simulink model "carsim_test2017"  (R2017b)
settings: Solver=FixedStepAuto  StartTime=0.0  StopTime=20  FixedStep=0.001  RelTol=1e-3
undefined symbols (not defined in the file or in its folder): ACC_MAP, ACC_MAP_ACCPEDL_BPY, ACC_MAP_REFSPD_BPX, BRK_MAP, BRK_MAP_BRKPEDL_BPX, ConvGear, CORNERING_STIFFNESS_APT, DIST_FR_AXLE_TO_CG_NVV, DIST_RE_AXLE_TO_CG_NVV, Fz, Fz_BPX, geartar, HYD_RATIO_APT, HYDRATIO_REFSPD_BPX, REFSPD_Q, REFSPD_R_LGT, REFSPD_R_WHL, STATIC_SPD, STATIC_TIME, VEHICLE_MASS_NVV, VEHICLE_YAW_INERTIA_NVV
libraries: simulink x22, simulink_extras x2, Solver_SF x1, SignalEditorBlockLib x1
(part 2 of 2)

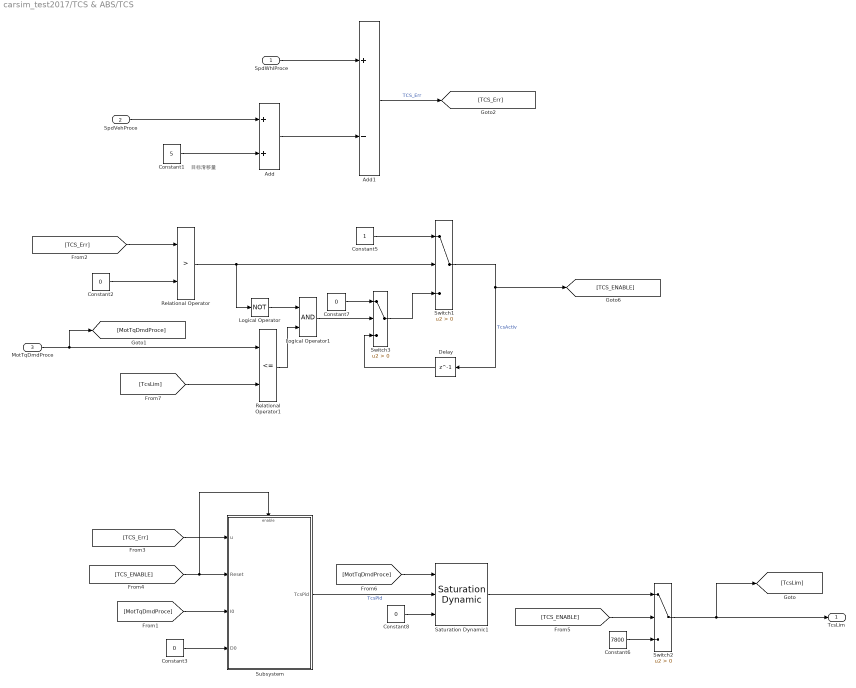
== system carsim_test2017/TCS & ABS/TCS ==
  note: 目标滑移量
  SpdWhlProce : Inport
  SpdVehProce : Inport  Port=2
  MotTqDmdProce : Inport  Port=3
  Add : Sum
  Add1 : Sum  Inputs=+-
  Constant1 : Constant  Value=5
  Constant{2..3,7..8} (4 alike) : Constant  Value=0
  Constant5 : Constant
  Constant6 : Constant  Value=7800
  Delay : Delay  DelayLength=1
  Logical Operator : Logic  Operator=NOT  AllPortsSameDT=off  OutDataTypeStr=boolean
  Logical Operator1 : Logic  AllPortsSameDT=off  OutDataTypeStr=boolean
  Relational Operator : RelationalOperator  Operator=>  OutDataTypeStr=boolean  RndMeth=Simplest
  Relational Operator1 : RelationalOperator  Operator=<=  OutDataTypeStr=boolean  RndMeth=Simplest
  Saturation Dynamic1 : simulink/Discontinuities/Saturation Dynamic  OutMin=[]  OutMax=[]  OutDataTypeStr=Inherit: Same as second input  OutDataType=fixdt(1, 16)  OutScaling=2^-10  DoSatur=off
  Subsystem : Subsystem
  Switch1 : Switch  Criteria=u2 > Threshold
  Switch2 : Switch  Criteria=u2 > Threshold
  Switch3 : Switch  Criteria=u2 > Threshold
  TcsLim : Outport
  wires:
  [TCS_Err] -> Subsystem/1(u)
  Constant5/1 -> Switch1/1
  Switch1/1 -> [TCS_ENABLE], Delay/1  "TcsActiv"
  [MotTqDmdProce] -> Saturation Dynamic1/1
  [TCS_ENABLE] -> Subsystem/Enable, Subsystem/2(Reset)
  Switch2/1 -> TcsLim/1, [TcsLim]
  Logical Operator/1 -> Logical Operator1/1
  Add/1 -> Add1/2
  [TcsLim] -> Relational Operator1/2
  Constant2/1 -> Relational Operator/2
  Switch3/1 -> Switch1/3
  Constant8/1 -> Saturation Dynamic1/3
  Logical Operator1/1 -> Switch3/2
  Add1/1 -> [TCS_Err]  "TCS_Err"
  Constant1/1 -> Add/2
  Delay/1 -> Switch3/3
  MotTqDmdProce/1 -> [MotTqDmdProce], Relational Operator1/1
  Relational Operator1/1 -> Logical Operator1/2
  Subsystem/1(TcsPid) -> Saturation Dynamic1/2  "TcsPid"
  Relational Operator/1 -> Logical Operator/1, Switch1/2
  SpdWhlProce/1 -> Add1/1
  [TCS_ENABLE] -> Switch2/2
  Constant7/1 -> Switch3/1
  [TCS_Err] -> Relational Operator/1
  Constant6/1 -> Switch2/3
  Saturation Dynamic1/1 -> Switch2/1
  [MotTqDmdProce] -> Subsystem/3(I0)
  Constant3/1 -> Subsystem/4(D0)
  SpdVehProce/1 -> Add/1

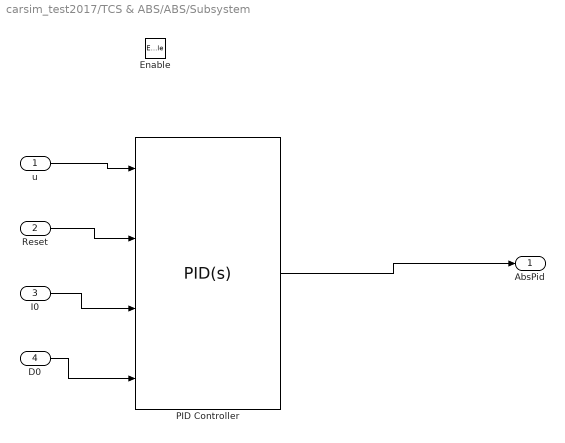
== system carsim_test2017/TCS & ABS/ABS/Subsystem ==
  u : Inport
  Reset : Inport  Port=2
  I0 : Inport  Port=3
  D0 : Inport  Port=4
  Enable : EnablePort  StatesWhenEnabling=reset
  PID Controller : simulink/Continuous/PID Controller  Controller=PID  Form=Parallel  TimeDomain=Continuous-time  SampleTime=-1  IntegratorMethod=Forward Euler  ControllerParametersSource=internal  P=100  I=500  D=0  N=100  UseFilter=on  TunerSelectOption=Transfer Function Based (PID Tuner App)  InitialConditionSource=external  InitialConditionForIntegrator=0  InitialConditionForFilter=0  DifferentiatorICPrevScaledInput=0  ExternalReset=either  TrackingMode=off  Kt=1  LimitOutput=off  UpperSaturationLimit=inf  LowerSaturationLimit=-inf  LinearizeAsGain=on  AntiWindupMode=none  Kb=1  POutMin=[]  POutMax=[]  IOutMin=[]  IOutMax=[]  DOutMin=[]  DOutMax=[]  NOutMin=[]  NOutMax=[]  SumOutMin=[]  SumOutMax=[]  SaturationOutMin=[]  SaturationOutMax=[]  PParamMin=[]  PParamMax=[]  IParamMin=[]  IParamMax=[]  DParamMin=[]  DParamMax=[]  NParamMin=[]  NParamMax=[]  KbParamMin=[]  KbParamMax=[]  KtParamMin=[]  KtParamMax=[]  KbOutMin=[]  KbOutMax=[]  KtOutMin=[]  KtOutMax=[]  IntegratorOutMin=[]  IntegratorOutMax=[]  FilterOutMin=[]  FilterOutMax=[]  SumI1OutMin=[]  SumI1OutMax=[]  SumI2OutMin=[]  SumI2OutMax=[]  SumI3OutMin=[]  SumI3OutMax=[]  SumDOutMin=[]  SumDOutMax=[]  DifferentiatorOutMin=[]  DifferentiatorOutMax=[]  FilterDiffOutCoefMin=[]  FilterDiffOutCoefMax=[]  ReciprocalOutMin=[]  ReciprocalOutMax=[]  SumDenOutMin=[]  SumDenOutMax=[]  SumNumOutMin=[]  SumNumOutMax=[]  DivideOutMin=[]  DivideOutMax=[]  IntegratorContinuousStateAttributes=''  IntegratorStateMustResolveToSignalObject=off  IntegratorRTWStateStorageClass=Auto  FilterContinuousStateAttributes=''  FilterStateMustResolveToSignalObject=off  FilterRTWStateStorageClass=Auto  InitialConditionSetting=State (most efficient)
  AbsPid : Outport  OutputWhenDisabled=reset  InitialOutput=-8000
  wires:
  Reset/1 -> PID Controller/2
  I0/1 -> PID Controller/3
  PID Controller/1 -> AbsPid/1
  u/1 -> PID Controller/1
  D0/1 -> PID Controller/4

== system carsim_test2017/TCS & ABS/TCS/Subsystem ==
  u : Inport
  Reset : Inport  Port=2
  I0 : Inport  Port=3
  D0 : Inport  Port=4
  Enable : EnablePort  StatesWhenEnabling=reset
  PID Controller : simulink/Continuous/PID Controller  Controller=PID  Form=Parallel  TimeDomain=Continuous-time  SampleTime=-1  IntegratorMethod=Forward Euler  ControllerParametersSource=internal  P=-100  I=-500  D=0  N=100  UseFilter=on  TunerSelectOption=Transfer Function Based (PID Tuner App)  InitialConditionSource=external  InitialConditionForIntegrator=0  InitialConditionForFilter=0  DifferentiatorICPrevScaledInput=0  ExternalReset=either  TrackingMode=off  Kt=1  LimitOutput=off  UpperSaturationLimit=inf  LowerSaturationLimit=-inf  LinearizeAsGain=on  AntiWindupMode=none  Kb=1  POutMin=[]  POutMax=[]  IOutMin=[]  IOutMax=[]  DOutMin=[]  DOutMax=[]  NOutMin=[]  NOutMax=[]  SumOutMin=[]  SumOutMax=[]  SaturationOutMin=[]  SaturationOutMax=[]  PParamMin=[]  PParamMax=[]  IParamMin=[]  IParamMax=[]  DParamMin=[]  DParamMax=[]  NParamMin=[]  NParamMax=[]  KbParamMin=[]  KbParamMax=[]  KtParamMin=[]  KtParamMax=[]  KbOutMin=[]  KbOutMax=[]  KtOutMin=[]  KtOutMax=[]  IntegratorOutMin=[]  IntegratorOutMax=[]  FilterOutMin=[]  FilterOutMax=[]  SumI1OutMin=[]  SumI1OutMax=[]  SumI2OutMin=[]  SumI2OutMax=[]  SumI3OutMin=[]  SumI3OutMax=[]  SumDOutMin=[]  SumDOutMax=[]  DifferentiatorOutMin=[]  DifferentiatorOutMax=[]  FilterDiffOutCoefMin=[]  FilterDiffOutCoefMax=[]  ReciprocalOutMin=[]  ReciprocalOutMax=[]  SumDenOutMin=[]  SumDenOutMax=[]  SumNumOutMin=[]  SumNumOutMax=[]  DivideOutMin=[]  DivideOutMax=[]  IntegratorContinuousStateAttributes=''  IntegratorStateMustResolveToSignalObject=off  IntegratorRTWStateStorageClass=Auto  FilterContinuousStateAttributes=''  FilterStateMustResolveToSignalObject=off  FilterRTWStateStorageClass=Auto  InitialConditionSetting=State (most efficient)
  TcsPid : Outport  OutputWhenDisabled=reset  InitialOutput=7800
  wires:
  D0/1 -> PID Controller/4
  u/1 -> PID Controller/1
  PID Controller/1 -> TcsPid/1
  I0/1 -> PID Controller/3
  Reset/1 -> PID Controller/2

== matlab function carsim_test2017/Subsystem/MATLAB Function1 ==
  data: a11 input; A output; a12 input; a21 input; a22 input
function A = fcn(a11, a12, a21, a22)
%#codegen
A = [a11, a12; a21, a22];
end

== matlab function carsim_test2017/Subsystem/MATLAB Function ==
  data: x input; dx output; u input; y output; A input; B input; C input; D input
function [dx, y] = state_space_derivative(x, u, A, B, C, D)
    % 计算连续时间状态导数
    dx = A * x + B * u;
    y  = C * x + D * u;
end

== matlab function carsim_test2017/Subsystem/MATLAB Function2 ==
  data: b11 input; B output; b21 input
function B = fcn(b11, b21)
%#codegen
B = [b11;b21];
end

== matlab function carsim_test2017/Subsystem/MATLAB Function3 ==
  data: a11 input; A output; a12 input; a21 input; a22 input
function A = fcn(a11, a12, a21, a22)
%#codegen
A = [a11, a12; a21, a22];
end

== matlab function carsim_test2017/Subsystem/MATLAB Function4 ==
  data: b11 input; B output; b21 input
function B = fcn(b11, b21)
%#codegen
B = [b11;b21];
end

== matlab function carsim_test2017/MATLAB Function ==
  data: a_meas input; omega_pitch input; v_wheel input; is_static input; dt input; Q input; R_wheel input; R_accel input; v output; b output; theta output; a output; P output
function [v, b, theta, a, P] = vehicleSpeedEKF4(a_meas, omega_pitch, v_wheel, is_static, dt, Q, R_wheel, R_accel)
% vehicleSpeedEKF4 - 四维EKF车速估计（增加真实加速度状态）
%
% 输入:
%   a_meas      - 纵向加速度计测量值 (m/s^2)
%   omega_pitch - 俯仰角速度 (rad/s)
%   v_wheel     - 轮速等效车速 (m/s)
%   is_static   - 静止标志 (true/false)
%   dt          - 采样时间 (s)
%   Q           - 过程噪声协方差 (4×4)
%   R_wheel     - 轮速观测噪声方差 (标量)
%   R_accel     - 加速度计观测噪声方差 (标量)
%
% 输出:
%   v, b, theta, a - 估计的状态
%   P             - 误差协方差矩阵 (4×4)
%
% 内部常量（可修改）：
%   R_STAT_V  - 静止时虚拟速度零观测噪声 (默认 1e-4)
%   R_STAT_A  - 静止时加速度计观测噪声 (默认 0.01)
%
% 重置滤波器: clear vehicleSpeedEKF4

    persistent x P_persistent
    g = 9.81;
    
    % 静止观测噪声（内部固定）
    R_STAT_V = 1e-6;
    R_STAT_A = 0.01;
    
    % 初始化
    if isempty(x)
        x = [0; 0; 0; 0];                     % [v; b; theta; a]
        P_persistent = diag([1, 0.1, 0.01, 1]); % 初始协方差
    end
    
    % ========== 预测 ==========
    v_prev = x(1); b_prev = x(2); theta_prev = x(3); a_prev = x(4);
    
    % 状态预测（非线性部分仅theta）
    v_pred   = v_prev + a_prev * dt;
    b_pred   = b_prev;
    theta_pred = theta_prev + omega_pitch * dt;
    a_pred   = a_prev;
    x_pred = [v_pred; b_pred; theta_pred; a_pred];
    
    % 雅可比矩阵 F (4×4)
    F = [1, 0, 0, dt;
         0, 1, 0, 0;
         0, 0, 1, 0;
         0, 0, 0, 1];
    
    P_pred = F * P_persistent * F' + Q;
    
    % ========== 更新 ==========
    if is_static
        % 静止：观测 [0; a_meas]
        z_pred = [v_pred; b_pred + g * sin(theta_pred)];
        z = [0; a_meas];
        H = [1, 0, 0, 0;
             0, 1, g*cos(theta_pred), 0];
        R = diag([R_STAT_V, R_STAT_A]);
    else
        % 运动：观测 [v_wheel; a_meas]
        z_pred = [v_pred; a_pred + b_pred + g * sin(theta_pred)];
        z = [v_wheel; a_meas];
        H = [1, 0, 0, 0;
             0, 1, g*cos(theta_pred), 1];
        R = diag([R_wheel, R_accel]);
    end
    
    % 卡尔曼更新
    y = z - z_pred;
    S = H * P_pred * H' + R;
    K = P_pred * H' / S;
    x = x_pred + K * y;
    P_persistent = (eye(4) - K * H) * P_pred;
    
    % 输出
    v = x(1);
    b = x(2);
    theta = x(3);
    a = x(4);
    P = P_persistent;
end

== matlab function carsim_test2017/Subsystem1/MATLAB Function ==
  data: slipFlags input; wheelSpeedOut output; wheelSpeeds input; allSlipFlag output
function [wheelSpeedOut, allSlipFlag] = computeWheelSpeed(slipFlags, wheelSpeeds)
%#codegen
% computeWheelSpeed: output mean of non-slip wheel speeds, or min if all slip.
%
% Inputs:
%   slipFlags   - slip indicator array (0 = no slip, nonzero = slip)
%   wheelSpeeds - wheel speed array (same number of elements as slipFlags)
%
% Outputs:
%   wheelSpeedOut - calculated wheel speed
%   allSlipFlag   - 1 (double) if all wheels are slipping, 0 (double) otherwise

    % Check that both inputs have the same total number of elements
    if numel(slipFlags) ~= numel(wheelSpeeds)
        error('slipFlags and wheelSpeeds must have the same number of elements.');
    end

    % Convert to logical array (0 -> false, nonzero -> true)
    slipLogical = logical(slipFlags);

    % Determine if all wheels are slipping, and store directly as double (0 or 1)
    % This avoids changing the variable type later, satisfying code generation.
    allSlipFlag = double(all(slipLogical(:)));

    if allSlipFlag
        % All wheels slip: output the minimum wheel speed
        wheelSpeedOut = min(wheelSpeeds(:));
    else
        % Some wheels not slipping: output mean of those speeds
        % Logical indexing uses linear order (column-major), works for any shape
        wheelSpeedOut = mean(wheelSpeeds(~slipLogical));
    end
end

== matlab function carsim_test2017/MATLAB Function1 ==
  data: u input; y output; Ts input; delay input
function y = turnOnDelay(u, Ts,  delay)
%#codegen
% turnOnDelay - Turn-on delay for multidimensional input (no partial assignment)
%
%   Inputs:
%       u     : current input (any dimension, nonzero = true)
%       Ts    : sample time in seconds (must be > 0)
%       delay : delay time in seconds (>= 0)
%   Output:
%       y     : delayed output (same size as u, double 0 or 1)

persistent timerCount lastInput output delaySteps

% ---------- Validate Ts ----------
if Ts <= 0
    error('Sample time Ts must be greater than 0.');
end

% ---------- Initialize persistent states ----------
if isempty(timerCount)
    timerCount = zeros(size(u));
    lastInput  = false(size(u));
    output     = false(size(u));
    delaySteps = max(0, round(delay / Ts));
else
    % If input size changes, reinitialize
    if ~isequal(size(timerCount), size(u))
        timerCount = zeros(size(u));
        lastInput  = false(size(u));
        output     = false(size(u));
        delaySteps = max(0, round(delay / Ts));
    end
end

% Update delay steps if parameters changed online
newSteps = max(0, round(delay / Ts));
if newSteps ~= delaySteps
    delaySteps = newSteps;
end

% ---------- Current input as logical ----------
currentInput = (u ~= 0);

% ---------- Detect edges ----------
rise = currentInput & ~lastInput;   % 0→1 transition
hold = currentInput & ~rise;        % stayed 1 (not just rose)

% ---------- Update per‑channel timers (completely index‑free) ----------
% Timer logic:
%   - on rising edge: reset to 0
%   - if input stays true: increment by 1
%   - if input false: reset to 0
% Arithmetic equivalent (elementwise):
%   timerCount = (timerCount .* ~rise + hold) .* currentInput;
% But we must also handle the case when delaySteps becomes 0 (no delay),
% then output should be true immediately for rising edge? Original behavior
% says: rising edge sets timer=0, and if delaySteps=0 output goes true only
% after one sample (because on the rising sample, output remains false).
% Our arithmetic does exactly that.

timerCount = (timerCount .* (~rise) + hold) .* currentInput;

% ---------- Compute output completely by elementwise logic ----------
% Output true only when input is true, NOT on the rising edge, and timer >= delaySteps.
% Since 'hold' already excludes the rising edge, we can simply use:
output = hold & (timerCount >= delaySteps);

% ---------- Store current input for next step ----------
lastInput = currentInput;

% ---------- Output ----------
y = double(output);
end

== matlab function carsim_test2017/Subsystem1/MATLAB Function1 ==
  data: u input; y output; Ts input; delay input
function y = turnOnDelay(u, Ts, delay)
%#codegen
% turnOnDelay - Turn-on delay for multidimensional input (no partial assignment)
%
%   Inputs:
%       u     : current input (any dimension, nonzero = true)
%       Ts    : sample time in seconds (must be > 0)
%       delay : delay time in seconds (>= 0)
%   Output:
%       y     : delayed output (same size as u, double 0 or 1)

persistent timerCount lastInput output delaySteps

% ---------- Validate Ts ----------
if Ts <= 0
    error('Sample time Ts must be greater than 0.');
end

% ---------- Initialize persistent states ----------
if isempty(timerCount)
    timerCount = zeros(size(u));
    lastInput  = false(size(u));
    output     = false(size(u));
    delaySteps = max(0, round(delay / Ts));
else
    % If input size changes, reinitialize
    if ~isequal(size(timerCount), size(u))
        timerCount = zeros(size(u));
        lastInput  = false(size(u));
        output     = false(size(u));
        delaySteps = max(0, round(delay / Ts));
    end
end

% Update delay steps if parameters changed online
newSteps = max(0, round(delay / Ts));
if newSteps ~= delaySteps
    delaySteps = newSteps;
end

% ---------- Current input as logical ----------
currentInput = (u ~= 0);

% ---------- Detect edges ----------
rise = currentInput & ~lastInput;   % 0→1 transition
hold = currentInput & ~rise;        % stayed 1 (not just rose)

% ---------- Update per‑channel timers (completely index‑free) ----------
% Timer logic:
%   - on rising edge: reset to 0
%   - if input stays true: increment by 1
%   - if input false: reset to 0
% Arithmetic equivalent (elementwise):
%   timerCount = (timerCount .* ~rise + hold) .* currentInput;
% But we must also handle the case when delaySteps becomes 0 (no delay),
% then output should be true immediately for rising edge? Original behavior
% says: rising edge sets timer=0, and if delaySteps=0 output goes true only
% after one sample (because on the rising sample, output remains false).
% Our arithmetic does exactly that.

timerCount = (timerCount .* (~rise) + hold) .* currentInput;

% ---------- Compute output completely by elementwise logic ----------
% Output true only when input is true, NOT on the rising edge, and timer >= delaySteps.
% Since 'hold' already excludes the rising edge, we can simply use:
output = hold & (timerCount >= delaySteps);

% ---------- Store current input for next step ----------
lastInput = currentInput;

% ---------- Output ----------
y = double(output);
end

== matlab function carsim_test2017/Subsystem1/MATLAB Function2 ==
  data: u input; y output; Ts input; delay input
function y = turnOnDelay(u, Ts, delay)
%#codegen
% turnOnDelay - Turn-on delay for multidimensional input (no partial assignment)
%
%   Inputs:
%       u     : current input (any dimension, nonzero = true)
%       Ts    : sample time in seconds (must be > 0)
%       delay : delay time in seconds (>= 0)
%   Output:
%       y     : delayed output (same size as u, double 0 or 1)

persistent timerCount lastInput output delaySteps

% ---------- Validate Ts ----------
if Ts <= 0
    error('Sample time Ts must be greater than 0.');
end

% ---------- Initialize persistent states ----------
if isempty(timerCount)
    timerCount = zeros(size(u));
    lastInput  = false(size(u));
    output     = false(size(u));
    delaySteps = max(0, round(delay / Ts));
else
    % If input size changes, reinitialize
    if ~isequal(size(timerCount), size(u))
        timerCount = zeros(size(u));
        lastInput  = false(size(u));
        output     = false(size(u));
        delaySteps = max(0, round(delay / Ts));
    end
end

% Update delay steps if parameters changed online
newSteps = max(0, round(delay / Ts));
if newSteps ~= delaySteps
    delaySteps = newSteps;
end

% ---------- Current input as logical ----------
currentInput = (u ~= 0);

% ---------- Detect edges ----------
rise = currentInput & ~lastInput;   % 0→1 transition
hold = currentInput & ~rise;        % stayed 1 (not just rose)

% ---------- Update per‑channel timers (completely index‑free) ----------
% Timer logic:
%   - on rising edge: reset to 0
%   - if input stays true: increment by 1
%   - if input false: reset to 0
% Arithmetic equivalent (elementwise):
%   timerCount = (timerCount .* ~rise + hold) .* currentInput;
% But we must also handle the case when delaySteps becomes 0 (no delay),
% then output should be true immediately for rising edge? Original behavior
% says: rising edge sets timer=0, and if delaySteps=0 output goes true only
% after one sample (because on the rising sample, output remains false).
% Our arithmetic does exactly that.

timerCount = (timerCount .* (~rise) + hold) .* currentInput;

% ---------- Compute output completely by elementwise logic ----------
% Output true only when input is true, NOT on the rising edge, and timer >= delaySteps.
% Since 'hold' already excludes the rising edge, we can simply use:
output = hold & (timerCount >= delaySteps);

% ---------- Store current input for next step ----------
lastInput = currentInput;

% ---------- Output ----------
y = double(output);
end

== matlab function carsim_test2017/MATLAB Function2 ==
  data: gyro input; accel input; v_wheel input; dt input; v_car output; slip_flag input; a_long output; pitch_deg output
function [v_car, a_long, pitch_deg] = estimateVelocity(gyro, accel, v_wheel, dt, slip_flag)
% 基于单轮速+IMU的车速估计（修正版：雅可比矩阵修正，四元数归一化）
% 输入：
%   gyro      : 车体系三轴角速度 [wx;wy;wz] (rad/s)
%   accel     : 车体系三轴加速度 [ax;ay;az] (m/s^2)
%   v_wheel   : 后轴（或单个）轮速线速度 (m/s)
%   dt        : 时间步长 (s)
%   slip_flag : 打滑标志，0=正常，1=轮速不可信（噪声极大）
% 输出：
%   v_car     : 估计的前向车速 (m/s)
%   a_long    : 纵向运动加速度（不含重力分量）(m/s^2)
%   pitch_deg : 俯仰角（上坡为正，度）

    persistent kf
    if isempty(kf)
        kf = initializeFilter();
    end

    x = kf.x;
    P = kf.P;
    dx = kf.dx;
    mem = kf.mem;
    cfg = kf.cfg;

    % ---------- 1. 预测 ----------
    gW = [0; 0; -cfg.g];
    b_g = x(11:13);
    b_a = x(14:16);
    gyro_ub  = gyro - b_g;
    accel_ub = accel - b_a;

    R_BW = quat2rot(x(7:10));
    dq = rotvec2quat(gyro_ub * dt);
    q_BW_new = quatMul(x(7:10), dq);
    q_BW_new = normalizeQuat(q_BW_new);  % 归一化
    R_new = quat2rot(q_BW_new);

    acc_world = R_BW * accel_ub + gW;
    v_W_new = x(4:6) + acc_world * dt;
    p_W_new = x(1:3) + x(4:6)*dt + 0.5*acc_world*dt^2;
    x_new = [p_W_new; v_W_new; q_BW_new; b_g; b_a];

    % ---------- 2. 协方差预测 ----------
    Omega_x = skew(gyro_ub);
    A_x = skew(accel_ub);
    F = zeros(15);
    F(1:3,1:3)   = -Omega_x;
    F(1:3,10:12) = -eye(3);
    F(4:6,1:3)   = -R_BW * A_x;
    F(4:6,13:15) = -R_BW;
    F(7:9,4:6)   = eye(3);

    G = zeros(15,12);
    G(1:3,1:3)   = -eye(3);
    G(4:6,4:6)   = -R_BW;
    G(10:12,7:9) = eye(3);
    G(13:15,10:12)= eye(3);

    Qc = blkdiag(cfg.sigma_g^2*eye(3), cfg.sigma_a^2*eye(3), ...
                 cfg.sigma_bg^2*eye(3), cfg.sigma_ba^2*eye(3));
    Phi = eye(15) + F * dt;
    P_new = Phi * P * Phi' + Phi * G * Qc * G' * Phi' * dt;

    % ---------- 3. 观测更新 ----------
    function injectAndReset()
        x_new(7:10) = quatMul(x_new(7:10), rotvec2quat(dx(1:3)));
        x_new(7:10) = normalizeQuat(x_new(7:10));
        x_new(4:6)  = x_new(4:6)  + dx(4:6);
        x_new(1:3)  = x_new(1:3)  + dx(7:9);
        x_new(11:13)= x_new(11:13)+ dx(10:12);
        x_new(14:16)= x_new(14:16)+ dx(13:15);
        dx = zeros(15,1);
        R_new = quat2rot(x_new(7:10));
        v_W_new = x_new(4:6);
    end

    % 预计算车体系速度和重力向量（雅可比修正依赖）
    v_body = R_new' * v_W_new;
    g_body = R_new' * gW;

    % 3.1 轮速观测
    h_vx = v_body(1);
    H_vx = zeros(1,15);
    % 修正：用 v_body 构造反对称矩阵的对应行
    H_vx(1:3) = [0, -v_body(3), v_body(2)];
    H_vx(4:6) = R_new(:,1)';

    if slip_flag
        R_vx = 1e6;
    else
        if mem.wheel_init && dt > 0
            a_wheel_est = (v_wheel - mem.last_v_wheel)/dt;
            % 注意：此处 a_imu_est 是车体系 x 向的运动加速度（世界加速度投影）
            a_imu_est   = R_new(:,1)' * (R_new * accel_ub + gW);
            slip_factor = abs(a_wheel_est - a_imu_est);
            R_vx = cfg.sigma_vx_base * exp(cfg.slip_gain * slip_factor);
        else
            R_vx = cfg.sigma_vx_base;
            mem.wheel_init = true;
        end
    end
    mem.last_v_wheel = v_wheel;

    [P_new, dx] = ekfUpdate(P_new, dx, v_wheel - h_vx, H_vx, R_vx);
    injectAndReset();
    % 更新后需重新计算 v_body（因为速度/姿态更新）
    v_body = R_new' * v_W_new;

    % 3.2 侧向约束 vy=0
    h_vy = v_body(2);
    H_vy = zeros(1,15);
    H_vy(1:3) = [v_body(3), 0, -v_body(1)];
    H_vy(4:6) = R_new(:,2)';
    yaw_rate = gyro(3);
    if mem.yaw_init && dt > 0
        % 注意：侧滑检测逻辑可能需按车辆动力学修正，这里保留原逻辑框架
        slip_lat = abs((yaw_rate - mem.last_yaw_rate)/dt + accel(2));
    else
        slip_lat = 0;
        mem.yaw_init = true;
    end
    mem.last_yaw_rate = yaw_rate;
    R_vy = cfg.sigma_vy_base * exp(cfg.slip_gain_vy * slip_lat);
    [P_new, dx] = ekfUpdate(P_new, dx, 0 - h_vy, H_vy, R_vy);
    injectAndReset();
    v_body = R_new' * v_W_new;

    % 3.3 垂向约束 vz=0
    h_vz = v_body(3);
    H_vz = zeros(1,15);
    H_vz(1:3) = [-v_body(2), v_body(1), 0];
    H_vz(4:6) = R_new(:,3)';
    [P_new, dx] = ekfUpdate(P_new, dx, 0 - h_vz, H_vz, cfg.sigma_vz);
    injectAndReset();
    v_body = R_new' * v_W_new;
    g_body = R_new' * gW;

    % 3.4 重力对准
    if abs(norm(accel) - cfg.g) < cfg.grav_acc_thresh && norm(gyro) < cfg.grav_gyro_thresh
        z_grav = accel;
        h_grav = -g_body + x_new(14:16);
        H_grav = zeros(3,15);
        % 修正：使用 skew(g_body) 作为姿态误差的雅可比
        H_grav(1:3,1:3)   = skew(g_body);
        H_grav(1:3,13:15) = eye(3);
        [P_new, dx] = ekfUpdate(P_new, dx, z_grav - h_grav, H_grav, cfg.sigma_grav^2*eye(3));
        injectAndReset();
        v_body = R_new' * v_W_new;  % 不需要 g_body，但保持一致
    end

    % 3.5 零速更新
    if abs(v_wheel) < cfg.zupt_wheel_thresh && ...
       norm(accel - mem.last_accel) < cfg.zupt_accel_variation
        z_zupt = zeros(3,1);
        h_zupt = v_W_new;
        H_zupt = zeros(3,15);
        H_zupt(1:3,4:6) = eye(3);
        [P_new, dx] = ekfUpdate(P_new, dx, z_zupt - h_zupt, H_zupt, cfg.sigma_zupt^2*eye(3));
        injectAndReset();
    end
    mem.last_accel = accel;

    % ---------- 4. 保存状态 ----------
    kf.x = x_new;
    kf.P = P_new;
    kf.dx = dx;
    kf.mem = mem;

    % ---------- 5. 输出计算 ----------
    R_final = quat2rot(kf.x(7:10));
    v_body_final = R_final' * kf.x(4:6);
    v_car = v_body_final(1);

    % 纵向运动加速度（不含重力）
    b_a_final = kf.x(14:16);
    accel_ub_final = accel - b_a_final;
    a_body_motion = accel_ub_final + R_final' * gW;
    a_long = a_body_motion(1);

    % 俯仰角（度），上坡为正
    pitch = atan2(-R_final(3,1), sqrt(R_final(3,2)^2 + R_final(3,3)^2));
    pitch_deg = pitch * 180 / pi;
end

% ========== 初始化 ==========
function kf = initializeFilter()
    cfg = struct();
    cfg.g = 9.81;
    cfg.sigma_g = 0.01;
    cfg.sigma_a = 0.05;
    cfg.sigma_bg = 0.001;
    cfg.sigma_ba = 0.01;
    cfg.sigma_vx_base = 0.1;
    cfg.slip_gain = 10;
    cfg.sigma_vy_base = 1.0;
    cfg.slip_gain_vy = 5;
    cfg.sigma_vz = 1.0;
    cfg.sigma_grav = 0.2;
    cfg.grav_acc_thresh = 0.5;
    cfg.grav_gyro_thresh = 0.05;
    cfg.sigma_zupt = 0.01;
    cfg.zupt_wheel_thresh = 0.05;
    cfg.zupt_accel_variation = 0.1;

    x0 = zeros(16,1);
    x0(1:3) = [0;0;0];
    x0(4:6) = [0;0;0];
    x0(7:10) = [1;0;0;0];
    P0 = zeros(15);
    P0(1:3,1:3) = 0.01^2 * eye(3);
    P0(4:6,4:6) = 0.5^2 * eye(3);
    P0(7:9,7:9) = 0.5^2 * eye(3);
    P0(10:12,10:12) = 0.01^2 * eye(3);
    P0(13:15,13:15) = 0.05^2 * eye(3);

    mem.last_v_wheel = 0;
    mem.wheel_init   = false;
    mem.last_yaw_rate = 0;
    mem.yaw_init      = false;
    mem.last_accel    = zeros(3,1);

    kf.x = x0;
    kf.P = P0;
    kf.dx = zeros(15,1);
    kf.mem = mem;
    kf.cfg = cfg;
end

% ========== 工具函数 ==========
function R = quat2rot(q)
    q = q / norm(q);
    qw = q(1); qx = q(2); qy = q(3); qz = q(4);
    R = [1-2*(qy^2+qz^2), 2*(qx*qy - qz*qw), 2*(qx*qz + qy*qw);
         2*(qx*qy + qz*qw), 1-2*(qx^2+qz^2), 2*(qy*qz - qx*qw);
         2*(qx*qz - qy*qw), 2*(qy*qz + qx*qw), 1-2*(qx^2+qy^2)];
end

function q = quatMul(q1, q2)
    w1 = q1(1); x1 = q1(2); y1 = q1(3); z1 = q1(4);
    w2 = q2(1); x2 = q2(2); y2 = q2(3); z2 = q2(4);
    q = [w1*w2 - x1*x2 - y1*y2 - z1*z2;
         w1*x2 + x1*w2 + y1*z2 - z1*y2;
         w1*y2 - x1*z2 + y1*w2 + z1*x2;
         w1*z2 + x1*y2 - y1*x2 + z1*w2];
end

function q = normalizeQuat(q)
    q = q / norm(q);
end

function q = rotvec2quat(rotvec)
    angle = norm(rotvec);
    if angle < 1e-12
        q = [1;0;0;0];
    else
        axis = rotvec / angle;
        half = angle / 2;
        q = [cos(half); sin(half)*axis];
    end
end

function M = skew(v)
    M = [0, -v(3), v(2);
         v(3), 0, -v(1);
         -v(2), v(1), 0];
end

function [P, dx] = ekfUpdate(P, dx, y, H, R)
    S = H * P * H' + R;
    K = P * H' / S;
    dx = dx + K * y;
    P = (eye(size(P)) - K * H) * P;
end
